simulink library "HEV_Battery_Lib"  (R2024b)
settings: Solver=ode45  StartTime=0.0  StopTime=10.0  RelTol=1e-3  EnableMultiTasking=on
undefined symbols (not defined in the file or in its folder): HEV_Param, Hydride, Kt_Temps, Metal, Nickel
libraries: fl_lib x58, nesl_utility x31, $bdroot x12, Rcecm_lib x6, batteryecm_lib x3, Capacitors_lib x1, spsBatteryLib x1, simulink_extras x1, spsGroundLib x1, spsControlledCurrentSourceLib x1, spsVoltageMeasurementLib x1
(part 1 of 2)
Description:
  | Copyright 2014-2024 The MathWorks, Inc.
settings Model: Creator=smiller  LastModifiedBy=hcseu
settings SolverCC: AlgebraicLoopSolver=TrustRegion
settings DataIOCC: LimitDataPoints=on  SaveFormat=Array  SignalLoggingSaveFormat=ModelDataLogs  ReturnWorkspaceOutputs=off
settings OptimizationCC: ReuseModelBlockBuffer=off  ExpressionDepthLimit=2147483647  LifeSpan=inf
settings DebuggingCC: UnderspecifiedInitializationDetection=Classic  MergeDetectMultiDrivingBlocksExec=none  SolverPrmCheckMsg=warning  FcnCallInpInsideContextMsg=warning  UnconnectedInputMsg=warning  UnconnectedOutputMsg=warning  UnconnectedLineMsg=warning  AllowSymbolicDim=off  StateNameClashWarn=warning  PregeneratedLibrarySubsystemCodeDiagnostic=none  SFUnexpectedBacktrackingDiag=warning  SFNoUnconditionalDefaultTransitionDiag=warning  SFExecutionAtInitializationDiag=none  ArithmeticOperatorsInVariantConditions=warning
settings HardwareCC: ProdBitPerPointer=32  ProdBitPerSizeT=32  ProdBitPerPtrDiffT=32  ProdLargestAtomicFloat=None  ProdIntDivRoundTo=Undefined  ProdEndianess=Unspecified  ProdWordSize=32  ProdHWDeviceType=32-bit Generic
settings ModelReferenceCC: EnableRefExpFcnMdlSchedulingChecks=on  PropagateSignalLabelsOutOfModel=off
settings SFSimCC: SimUseLocalCustomCode=off  CustomCodeUndefinedFunction=UseInterfaceOnly
settings RTWCC: RTWUseLocalCustomCode=off  GPUComputeCapability=3.5  DLArmComputeVersion=19.05
settings CodeAppCC: StateflowObjectComments=on
settings GRTTargetCC: TargetLangStandard=C89/C90 (ANSI)  CombineOutputUpdateFcns=off  GRTInterface=on
settings ConfigComp: CovMetricSettings=dw  CovSaveCumulativeToWorkspaceVar=on  CovSaveSingleToWorkspaceVar=on  CovExternalEMLEnable=off  CovSFcnEnable=off

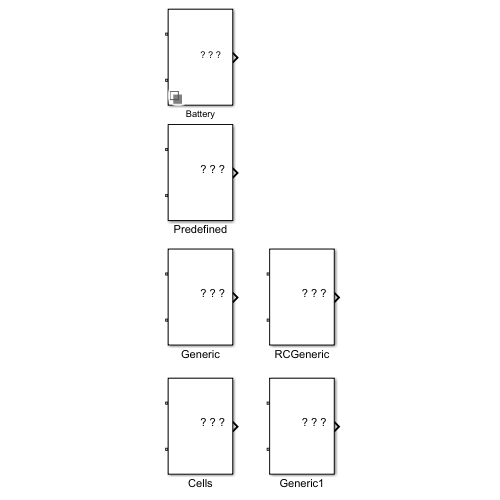
[thumbnail: Simulink's stored preview of the top-level diagram]
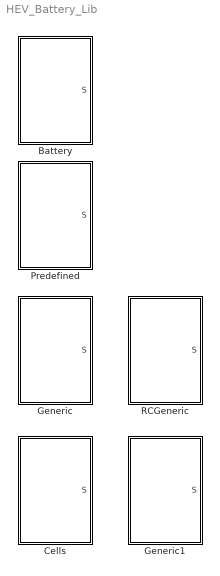
== system HEV_Battery_Lib ==
  Battery : Subsystem  BlockChoice=Predefined  Variant=on  VariantControlMode=label  LabelModeActiveChoice=Predefined
      mask Display:
      | blk = HEVPS_activeVariantBlock(gcb);
      | eval(get_param(blk, 'MaskDisplay'));
  Cells : Subsystem
      mask Display:
      | image(imread('HEV_Battery_Cells_IMAGE.jpg'));
      | port_label('LConn',1,'+');
      | port_label('LConn',2,'-');
      | port_label('output',1,'S');
  Generic : Subsystem
      mask Display:
      | image(imread('HEV_Battery_Custom_IMAGE.jpg'));
      | port_label('LConn',1,'+');
      | port_label('LConn',2,'-');
      | port_label('output',1,'S');
  Generic1 : Subsystem
      mask Display:
      | image(imread('HEV_Battery_Generic_IMAGE.jpg'));
      | port_label('LConn',1,'+');
      | port_label('LConn',2,'-');
      | port_label('output',1,'S');
  Predefined : Subsystem
      mask Display:
      | image(imread('HEV_Battery_Detailed_IMAGE.jpg'));
      | port_label('LConn',1,'+');
      | port_label('LConn',2,'-');
      | port_label('output',1,'S');
  RCGeneric : Subsystem
      mask Display:
      | image(imread('HEV_Battery_GenericRC_IMAGE.jpg'));
      | port_label('LConn',1,'+');
      | port_label('LConn',2,'-');
      | port_label('output',1,'S');

== system HEV_Battery_Lib/Battery ==
  Cells : $bdroot/Cells  SystemSampleTime=-1  VariantControl=Cells  VariantActivationTime=update diagram  AllowFlexibleInterface=on  Latency=0  AutoFrameSizeCalculation=off
  Generic : $bdroot/Generic  SystemSampleTime=-1  VariantControl=Generic  VariantActivationTime=update diagram  AllowFlexibleInterface=on  Latency=0  AutoFrameSizeCalculation=off
  Predefined : $bdroot/Predefined  SystemSampleTime=-1  VariantControl=Predefined  VariantActivationTime=update diagram  AllowFlexibleInterface=on  Latency=0  AutoFrameSizeCalculation=off
  + : PMIOPort  Side=Left
  - : PMIOPort  Port=2  Side=Left
  S : Outport  VectorParamsAs1DForOutWhenUnconnected=off

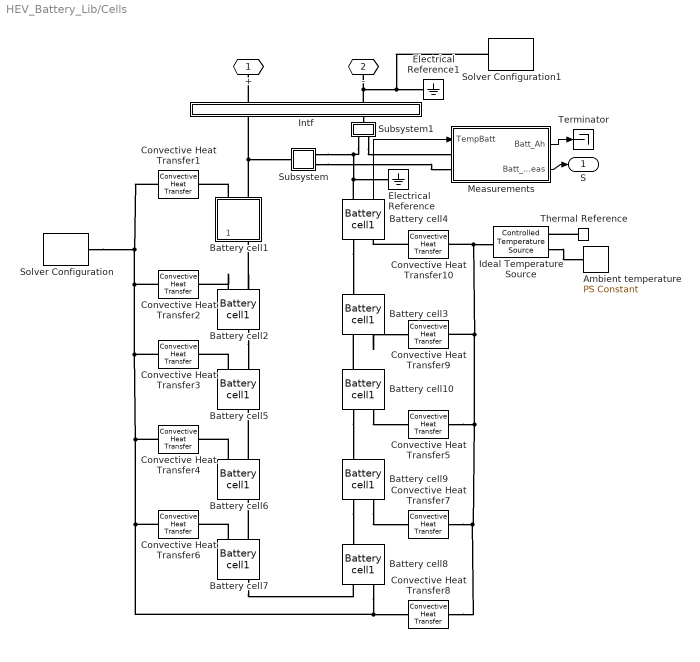
== system HEV_Battery_Lib/Cells ==
  Ambient temperature : fl_lib/Physical Signals/Sources/PS Constant  constant=273+25
  Battery cell1 : Subsystem
      mask Display:
      | % Battery icon
      | plot([1.5 0.4],[0 0])
      | plot(-[0.2 0.9 0.9 1.5],[0 0 -0.8 -0.8])
      | patch(([1 1 -1 -1]*0.15-0.5)*-1,[-1 1 1 -1]*0.4,[0;0;0]);
      | patch(([1 1 -1 -1]*0.15+0.1)*-1,[-1 1 1 -1]*0.9,[0;0;0]);
      | 
      | % Thermal port
      | plot([-0.5,-0.9],[1.2,1.2])
      | plot([-0.5,-0.9],[0.4,0.4])
      | plot([-0.9,-1.5],[0.8,0.8])
      | plot(-0.15*sin(0:2*pi/50:2*pi)-0.85,-0.35*cos(0:2*pi/50:2*pi)+0.8)
      | plot(0.15*sin(0:2*pi/50:pi)-0.55,-0.35*cos(0:2*pi/50:pi)+0.8)
      | 
      | % Plot points to set plot range
      | color('white');plot(1.5,1.5);plot(-1.5,-1.5)
      | 
      | color('red')
      | port_label('LConn',1,'H')
      | port_label('LConn',2,'+')
      | port_label('RConn',1,'-')
  Battery cell{2..10} (9 alike) : $bdroot/Cells/Battery cell1  SystemSampleTime=-1  VariantActivationTime=update diagram  AllowFlexibleInterface=on  Latency=0  AutoFrameSizeCalculation=off
  Convective Heat Transfer{1..10} (10 alike) : fl_lib/Thermal/Thermal Elements/Convective Heat Transfer  thermal_type=foundation.enum.constant_variable.constant  area=HEV_Param.Battery_Cell.Area m^2  heat_tr_coeff=HEV_Param.Battery_Cell.Rtheta W/(m^2 *K)  min_heat_tr_coeff=1e-3 W/(K*m^2)  T_specify=off  T_priority=High  T=0 K  T_nominal_specify=off  T_nominal_value=1  T_nominal_unit=K  Q_specify=off  Q_priority=High  Q=0 J/s  Q_nominal_specify=off  Q_nominal_value=1  Q_nominal_unit=J/s
  Electrical Reference : fl_lib/Electrical/Electrical Elements/Electrical Reference
  Electrical Reference1 : fl_lib/Electrical/Electrical Elements/Electrical Reference
  Ideal Temperature Source : fl_lib/Thermal/Thermal Sources/Controlled Temperature Source
  Intf : Subsystem  mask(Simscape Interface Element){T=100000}
      mask prompts: T "Pole in Transfer Function"
      mask help:
      | Ideal transformer between Simscape circuits.
      |
      | The Voltage across the two terminal pairs are equal and the current flowing through the two branches are equal.
      |
      | The coupling has a transfer function and you need to set the pole in the transfer function.
      mask Display:
      | %color('red');
      | %plot([0.3 0.7],[0.775 0.775]);
      | port_label('LConn', 1,'SPS1')
      | port_label('RConn', 1,'SS1')
      | color('black');
      | %plot([0.3 0.7],[0.225 0.225]);
      | port_label('LConn', 2,'SPS2')
      | port_label('RConn', 2,'SS2')
      | color('green')
      | %text(0.05,0.5,'I Src');
      | color('blue')
      | %text(0.75,0.5,'V Src');
  Measurements : Subsystem
  Solver Configuration : nesl_utility/Solver Configuration  PhysicalDomain=network_engine_domain  SubClassName=solver  LeftPortType=input  RightPortType=generic  Tones=[]  Harmonics=[]  SimulateNoise=off  Profile=off  UseLocalSampling=off  EnableSwitchedLinearOptims=on  FrequencyDomain=off  UseCCode=off  RelTol=0.001  AbsTol=0.001  MinStep=1e-09  ToWorkspace=off  RevertToSquareIcSolve=off  NumHomotopyIterations=100  PhasorMode=off  PhasorModeNumHarmonics=1  ConsistencySolver=NEWTON_XTOL_AFTER_FTOL  IndexReductionMethod=DerivativeReplacement  DoDC=off  ResidualTolerance=1e-09  ConsistencyTolSource=GLOBAL  ConsistencyAbsTol=0.001  ConsistencyRelTol=0.001  ConsistencyTolFactor=0.001  UseLocalSolver=on  LocalSolverChoice=NE_BACKWARD_EULER_ADVANCER  ResolveIndetEquations=on  FunctionEvalNumThread=1  LocalSolverSampleTime=0.001  DoFixedCost=off  MaxNonlinIter=3  MaxModeIter=2  ComputeImpulses=off  ImpulseIterations=2  LinearAlgebra=auto  LinearAlgebraNumThread=0  EquationFormulation=NE_TIME_EF  DelaysMemoryBudget=1024  AutomaticFiltering=on  FilteringTimeConstant=0.001  PartitionStorageMethod=AS_NEEDED  PartitionMemoryBudget=1024  PartitionMethod=ROBUST  MultibodyUseLocalSolver=off  MultibodyLocalSolverChoice=ODE1  MultibodyLocalSolverSampleTime=0.001
  Solver Configuration1 : nesl_utility/Solver Configuration  PhysicalDomain=network_engine_domain  SubClassName=solver  LeftPortType=input  RightPortType=generic  Tones=[]  Harmonics=[]  SimulateNoise=off  Profile=off  UseLocalSampling=off  EnableSwitchedLinearOptims=on  FrequencyDomain=off  UseCCode=off  RelTol=0.001  AbsTol=0.001  MinStep=1e-09  ToWorkspace=off  RevertToSquareIcSolve=off  NumHomotopyIterations=100  PhasorMode=off  PhasorModeNumHarmonics=1  ConsistencySolver=NEWTON_XTOL_AFTER_FTOL  IndexReductionMethod=DerivativeReplacement  DoDC=off  ResidualTolerance=1e-09  ConsistencyTolSource=GLOBAL  ConsistencyAbsTol=0.001  ConsistencyRelTol=0.001  ConsistencyTolFactor=0.001  UseLocalSolver=on  LocalSolverChoice=NE_BACKWARD_EULER_ADVANCER  ResolveIndetEquations=on  FunctionEvalNumThread=1  LocalSolverSampleTime=0.001  DoFixedCost=off  MaxNonlinIter=3  MaxModeIter=2  ComputeImpulses=off  ImpulseIterations=2  LinearAlgebra=auto  LinearAlgebraNumThread=0  EquationFormulation=NE_TIME_EF  DelaysMemoryBudget=1024  AutomaticFiltering=on  FilteringTimeConstant=0.001  PartitionStorageMethod=AS_NEEDED  PartitionMemoryBudget=1024  PartitionMethod=ROBUST  MultibodyUseLocalSolver=off  MultibodyLocalSolverChoice=ODE1  MultibodyLocalSolverSampleTime=0.001
  Subsystem : Subsystem
      mask Display: disp('S')
  Subsystem1 : Subsystem
      mask Display: disp('S');
  Terminator : Terminator
  Thermal Reference : fl_lib/Thermal/Thermal Elements/Thermal Reference
  + : PMIOPort  Side=Left
  - : PMIOPort  Port=2  Side=Left
  S : Outport  VectorParamsAs1DForOutWhenUnconnected=off
  wires:
  Measurements/2(Batt_Meas) -> S/1
  Measurements/1(Batt_Ah) -> Terminator/1
  Battery cell4/1 -> Measurements/1(TempBatt)
  connections:
  -/RConn1 -- Solver Configuration1/RConn1 -- Electrical Reference1/LConn1 -- Intf/RConn2
  Intf/RConn1 -- +/RConn1
  Intf/LConn2 -- Subsystem1/LConn1
  Subsystem1/RConn2 -- Measurements/LConn1
  Subsystem1/RConn1 -- Subsystem/RConn2 -- Battery cell4/RConn1 -- Electrical Reference/LConn1
  Subsystem/RConn1 -- Measurements/LConn2
  Battery cell1/LConn2 -- Subsystem/LConn1 -- Intf/LConn1
  Battery cell3/LConn1 -- Convective Heat Transfer9/RConn1
  Battery cell4/LConn2 -- Battery cell3/RConn1
  Battery cell2/LConn1 -- Convective Heat Transfer2/RConn1
  Battery cell1/LConn1 -- Convective Heat Transfer1/RConn1
  Ideal Temperature Source/RConn1 -- Ambient temperature/RConn1
  Thermal Reference/LConn1 -- Ideal Temperature Source/RConn2
  Battery cell10/LConn1 -- Convective Heat Transfer5/RConn1
  Battery cell10/RConn1 -- Battery cell3/LConn2
  Battery cell2/LConn2 -- Battery cell1/RConn1
  Convective Heat Transfer10/RConn1 -- Battery cell4/LConn1
  Convective Heat Transfer5/LConn1 -- Convective Heat Transfer7/LConn1 -- Convective Heat Transfer8/LConn1 -- Convective Heat Transfer9/LConn1 -- Convective Heat Transfer10/LConn1 -- Ideal Temperature Source/LConn1
  Battery cell6/LConn2 -- Battery cell5/RConn1
  Battery cell7/LConn2 -- Battery cell6/RConn1
  Battery cell9/LConn2 -- Battery cell8/RConn1
  Battery cell10/LConn2 -- Battery cell9/RConn1
  Battery cell7/RConn1 -- Battery cell8/LConn2
  Battery cell2/RConn1 -- Battery cell5/LConn2
  Battery cell5/LConn1 -- Convective Heat Transfer3/RConn1
  Battery cell6/LConn1 -- Convective Heat Transfer4/RConn1
  Battery cell7/LConn1 -- Convective Heat Transfer6/RConn1
  Battery cell9/LConn1 -- Convective Heat Transfer7/RConn1
  Convective Heat Transfer3/LConn1 -- Convective Heat Transfer4/LConn1 -- Convective Heat Transfer8/RConn1 -- Battery cell8/LConn1 -- Convective Heat Transfer6/LConn1 -- Convective Heat Transfer2/LConn1 -- Solver Configuration/RConn1 -- Convective Heat Transfer1/LConn1

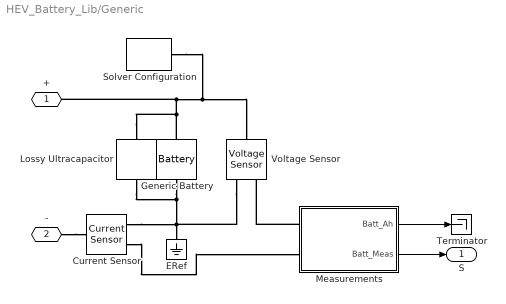
== system HEV_Battery_Lib/Generic ==
  Current Sensor : fl_lib/Electrical/Electrical Sensors/Current Sensor
  ERef : fl_lib/Electrical/Electrical Elements/Electrical Reference
  Generic Battery : batteryecm_lib/Battery  Vnom=HEV_Param.Battery_Sys.Nominal_Voltage V  prm_dir=1  R1_dis=2 Ohm  R1_ch=2 Ohm  R1=HEV_Param.Battery_Sys.Internal_Resistance Ohm  prm_AH=2  AH=HEV_Param.Battery_Sys.Rated_Capacity hr*A  V1=HEV_Param.Battery_Sys.Expn_Voltage V  AH1=HEV_Param.Battery_Sys.Expn_Charge hr*A  prm_R2=1  R2=2e+3 Ohm  Tmeas=298.15 K  charge_measurement_port=simscape.enum.battery.enable.no  prm_dyn=1  Rp1=0.005 Ohm  tau1=30 s  Rp2=0.005 Ohm  tau2=30 s  Rp3=0.005 Ohm  tau3=30 s  Rp4=0.005 Ohm  tau4=30 s  Rp5=0.005 Ohm  tau5=30 s  prm_fade=1  N_fade=100  AH_fade=45 hr*A  R1_fade=2.02 Ohm  R1_ch_fade=2.02 Ohm  V1_fade=10.35 V  prm_age=1  prm_age_OCV=1  OCV_age=0.9  SOC_age=60  Tmeas_age=298.15 K  delta_time_age_vec=[0] d  temperature_age_vec=[273] K  OCV_scaling_age=2.2134e6  OCV_offset_age=1.632e6  temp_exp_age=0.515833569 V  t_exp_age=0.75  Vnom_T2=12 V  R1_T2=2.2 Ohm  R1_T2_dis=2.2 Ohm  R1_T2_ch=2.2 Ohm  V1_T2=11.4 V  R2_T2=2200 Ohm  Rp1_T2=0.005 Ohm  tau1_T2=30 s  Rp2_T2=0.005 Ohm  tau2_T2=30 s  Rp3_T2=0.005 Ohm  tau3_T2=30 s  Rp4_T2=0.005 Ohm  tau4_T2=30 s  Rp5_T2=0.005 Ohm  tau5_T2=30 s  Tmeas2=273.15 K  thermal_port=simscape.enum.thermaleffects.omit  thermal_mass=30000 J/K  i_specify=off  i_priority=None  i=0 A  i_nominal_specify=off  i_nominal_value=1  i_nominal_unit=A  v_specify=off  v_priority=None  v=0 V  v_nominal_specify=off  v_nominal_value=1  v_nominal_unit=V  charge_specify=on  charge_priority=High  charge=HEV_Param.Battery_Sys.Initial_Charge hr*A  charge_nominal_specify=off  charge_nominal_value=1  charge_nominal_unit=A*hr  num_cycles_specify=off  num_cycles_priority=High  num_cycles=0  num_cycles_nominal_specify=off  num_cycles_nominal_value=1  num_cycles_nominal_unit=1  temperature_specify=off  temperature_priority=High  temperature=298.15 K  temperature_nominal_specify=off  temperature_nominal_value=1  temperature_nominal_unit=K
  Lossy Ultracapacitor : Capacitors_lib/Lossy Ultracapacitor  C0=HEV_Param.UltraCapacitor.Nominal_Capacitance F  Cv=HEV_Param.UltraCapacitor.Rate_C_V F/V  R=HEV_Param.UltraCapacitor.Series_R Ohm  Rd=HEV_Param.UltraCapacitor.Self_Discharge_R Ohm  i_specify=off  i_priority=High  i=0 A  i_nominal_specify=off  i_nominal_value=1  i_nominal_unit=A  vc_specify=off  vc_priority=High  vc=0 V  vc_nominal_specify=off  vc_nominal_value=1  vc_nominal_unit=V
      settings: InternalSimscapePortConfiguration="{\"Bottom\":[],\"Left\":[{\"id\":\"p\",\"label\":\"+\",\"type\":\"foundation.electrical.electrical\"}],\"Right\":[{\"id\":\"n\",\"label\":\"-\",\"type\":\"foundation.electrical.electrical\"}],\"Top\":[]}"
  Measurements : Subsystem
  Solver Configuration : nesl_utility/Solver Configuration  PhysicalDomain=network_engine_domain  SubClassName=solver  LeftPortType=input  RightPortType=generic  Tones=[]  Harmonics=[]  SimulateNoise=off  Profile=off  UseLocalSampling=off  EnableSwitchedLinearOptims=on  FrequencyDomain=off  UseCCode=off  RelTol=0.001  AbsTol=0.001  MinStep=1e-09  ToWorkspace=off  RevertToSquareIcSolve=off  NumHomotopyIterations=100  PhasorMode=off  PhasorModeNumHarmonics=1  ConsistencySolver=NEWTON_XTOL_AFTER_FTOL  IndexReductionMethod=DerivativeReplacement  DoDC=off  ResidualTolerance=1e-09  ConsistencyTolSource=GLOBAL  ConsistencyAbsTol=0.001  ConsistencyRelTol=0.001  ConsistencyTolFactor=0.001  UseLocalSolver=off  LocalSolverChoice=NE_BACKWARD_EULER_ADVANCER  ResolveIndetEquations=on  FunctionEvalNumThread=1  LocalSolverSampleTime=0.001  DoFixedCost=off  MaxNonlinIter=3  MaxModeIter=2  ComputeImpulses=off  ImpulseIterations=2  LinearAlgebra=auto  LinearAlgebraNumThread=0  EquationFormulation=NE_TIME_EF  DelaysMemoryBudget=1024  AutomaticFiltering=on  FilteringTimeConstant=0.001  PartitionStorageMethod=AS_NEEDED  PartitionMemoryBudget=1024  PartitionMethod=ROBUST  MultibodyUseLocalSolver=off  MultibodyLocalSolverChoice=ODE1  MultibodyLocalSolverSampleTime=0.001
  Terminator : Terminator
  Voltage Sensor : fl_lib/Electrical/Electrical Sensors/Voltage Sensor
  + : PMIOPort  Side=Left
  - : PMIOPort  Port=2  Side=Left
  S : Outport  VectorParamsAs1DForOutWhenUnconnected=off
  wires:
  Measurements/2(Batt_Meas) -> S/1
  Measurements/1(Batt_Ah) -> Terminator/1
  connections:
  -/RConn1 -- Current Sensor/LConn1
  Current Sensor/RConn1 -- Measurements/LConn2
  Lossy Ultracapacitor/RConn1 -- Current Sensor/RConn2 -- ERef/LConn1 -- Voltage Sensor/RConn2 -- Generic Battery/RConn1
  Lossy Ultracapacitor/LConn1 -- +/RConn1 -- Solver Configuration/RConn1 -- Voltage Sensor/LConn1 -- Generic Battery/LConn1
  Measurements/LConn1 -- Voltage Sensor/RConn1

== system HEV_Battery_Lib/Generic1 ==
  Current Sensor : fl_lib/Electrical/Electrical Sensors/Current Sensor
  Electrical Reference : fl_lib/Electrical/Electrical Elements/Electrical Reference
  Generic Battery : batteryecm_lib/Battery  Vnom=HEV_Param.Battery_Sys.Nominal_Voltage V  prm_dir=1  R1_dis=2 Ohm  R1_ch=2 Ohm  R1=HEV_Param.Battery_Sys.Internal_Resistance Ohm  prm_AH=2  AH=HEV_Param.Battery_Sys.Rated_Capacity hr*A  V1=HEV_Param.Battery_Sys.Expn_Voltage V  AH1=HEV_Param.Battery_Sys.Expn_Charge hr*A  prm_R2=1  R2=2e+3 Ohm  Tmeas=298.15 K  charge_measurement_port=simscape.enum.battery.enable.no  prm_dyn=1  Rp1=0.005 Ohm  tau1=30 s  Rp2=0.005 Ohm  tau2=30 s  Rp3=0.005 Ohm  tau3=30 s  Rp4=0.005 Ohm  tau4=30 s  Rp5=0.005 Ohm  tau5=30 s  prm_fade=1  N_fade=100  AH_fade=45 hr*A  R1_fade=2.02 Ohm  R1_ch_fade=2.02 Ohm  V1_fade=10.35 V  prm_age=1  prm_age_OCV=1  OCV_age=0.9  SOC_age=60  Tmeas_age=298.15 K  delta_time_age_vec=[0] d  temperature_age_vec=[273] K  OCV_scaling_age=2.2134e6  OCV_offset_age=1.632e6  temp_exp_age=0.515833569 V  t_exp_age=0.75  Vnom_T2=12 V  R1_T2=2.2 Ohm  R1_T2_dis=2.2 Ohm  R1_T2_ch=2.2 Ohm  V1_T2=11.4 V  R2_T2=2200 Ohm  Rp1_T2=0.005 Ohm  tau1_T2=30 s  Rp2_T2=0.005 Ohm  tau2_T2=30 s  Rp3_T2=0.005 Ohm  tau3_T2=30 s  Rp4_T2=0.005 Ohm  tau4_T2=30 s  Rp5_T2=0.005 Ohm  tau5_T2=30 s  Tmeas2=273.15 K  thermal_port=simscape.enum.thermaleffects.omit  thermal_mass=30000 J/K  i_specify=off  i_priority=None  i=0 A  i_nominal_specify=off  i_nominal_value=1  i_nominal_unit=A  v_specify=off  v_priority=None  v=0 V  v_nominal_specify=off  v_nominal_value=1  v_nominal_unit=V  charge_specify=on  charge_priority=High  charge=HEV_Param.Battery_Sys.Initial_Charge hr*A  charge_nominal_specify=off  charge_nominal_value=1  charge_nominal_unit=A*hr  num_cycles_specify=off  num_cycles_priority=High  num_cycles=0  num_cycles_nominal_specify=off  num_cycles_nominal_value=1  num_cycles_nominal_unit=1  temperature_specify=off  temperature_priority=High  temperature=298.15 K  temperature_nominal_specify=off  temperature_nominal_value=1  temperature_nominal_unit=K
  Measurements : Subsystem
  Terminator : Terminator
  Voltage Sensor1 : fl_lib/Electrical/Electrical Sensors/Voltage Sensor
  + : PMIOPort  Side=Left
  - : PMIOPort  Port=2  Side=Left
  S : Outport  VectorParamsAs1DForOutWhenUnconnected=off
  wires:
  Measurements/2(Batt_Meas) -> S/1
  Measurements/1(Batt_Ah) -> Terminator/1
  connections:
  -/RConn1 -- Current Sensor/LConn1
  Measurements/LConn2 -- Current Sensor/RConn1
  Current Sensor/RConn2 -- Electrical Reference/LConn1 -- Generic Battery/RConn1 -- Voltage Sensor1/RConn2
  +/RConn1 -- Generic Battery/LConn1 -- Voltage Sensor1/LConn1
  Measurements/LConn1 -- Voltage Sensor1/RConn1

== system HEV_Battery_Lib/Predefined ==
  Battery : spsBatteryLib/Battery  BatType=Nickel-Metal-Hydride  NomV=HEV_Param.Battery_Det.Nominal_Voltage  NomQ=HEV_Param.Battery_Det.Rated_Capacity  SOC=HEV_Param.Battery_Det.Initial_SOC  Batt_Tr=30  PresetModel=on  MaxQ=8.7231  MinV=150  FullV=235.5932  Dis_rate=1.62  R=0.24691  Normal_OP=7.7885  expZone="[216.9492          1.62]"
  Electrical Reference : fl_lib/Electrical/Electrical Elements/Electrical Reference
  GF1 : Subsystem
      mask Display: disp('GF')
  Ground : spsGroundLib/Ground  LConnTagsString=a
  Intf : Subsystem  mask(Power Systems ST - Simscape Interface Element){T=100000}
      mask prompts: T "Pole in Transfer Function"
      mask help:
      | Ideal transformer between a Simscape Power Systems ST circuit and a Simscape circuit.
      |
      | The Voltage across the two terminal pairs are equal and the current flowing through the two branches are equal.
      |
      | The coupling has a transfer function and you need to set the pole in the transfer function.
      mask Display:
      | %color('red');
      | %plot([0.3 0.7],[0.775 0.775]);
      | port_label('LConn', 1,'SPS1')
      | port_label('RConn', 1,'SS1')
      | color('black');
      | %plot([0.3 0.7],[0.225 0.225]);
      | port_label('LConn', 2,'SPS2')
      | port_label('RConn', 2,'SS2')
      | color('green')
      | %text(0.05,0.5,'I Src');
      | color('blue')
      | %text(0.75,0.5,'V Src');
  Solver Configuration : nesl_utility/Solver Configuration  PhysicalDomain=network_engine_domain  SubClassName=solver  LeftPortType=input  RightPortType=generic  Tones=[]  Harmonics=[]  SimulateNoise=off  Profile=off  UseLocalSampling=off  EnableSwitchedLinearOptims=on  FrequencyDomain=off  UseCCode=off  RelTol=0.001  AbsTol=0.001  MinStep=1e-09  ToWorkspace=off  RevertToSquareIcSolve=off  NumHomotopyIterations=100  PhasorMode=off  PhasorModeNumHarmonics=1  ConsistencySolver=NEWTON_XTOL_AFTER_FTOL  IndexReductionMethod=DerivativeReplacement  DoDC=off  ResidualTolerance=1e-09  ConsistencyTolSource=GLOBAL  ConsistencyAbsTol=0.001  ConsistencyRelTol=0.001  ConsistencyTolFactor=0.001  UseLocalSolver=off  LocalSolverChoice=NE_BACKWARD_EULER_ADVANCER  ResolveIndetEquations=on  FunctionEvalNumThread=1  LocalSolverSampleTime=0.001  DoFixedCost=off  MaxNonlinIter=3  MaxModeIter=2  ComputeImpulses=off  ImpulseIterations=2  LinearAlgebra=auto  LinearAlgebraNumThread=0  EquationFormulation=NE_TIME_EF  DelaysMemoryBudget=1024  AutomaticFiltering=on  FilteringTimeConstant=0.001  PartitionStorageMethod=AS_NEEDED  PartitionMemoryBudget=1024  PartitionMethod=ROBUST  MultibodyUseLocalSolver=off  MultibodyLocalSolverChoice=ODE1  MultibodyLocalSolverSampleTime=0.001
  + : PMIOPort  Side=Left
  - : PMIOPort  Port=2  Side=Left
  S : Outport  VectorParamsAs1DForOutWhenUnconnected=off
  wires:
  Battery/1 -> GF1/1(In1)
  GF1/1(Out1) -> S/1
  connections:
  Intf/RConn2 -- Solver Configuration/RConn1 -- Electrical Reference/LConn1 -- -/RConn1
  Intf/LConn2 -- Battery/LConn2 -- Ground/LConn1
  Battery/LConn1 -- Intf/LConn1
  +/RConn1 -- Intf/RConn1

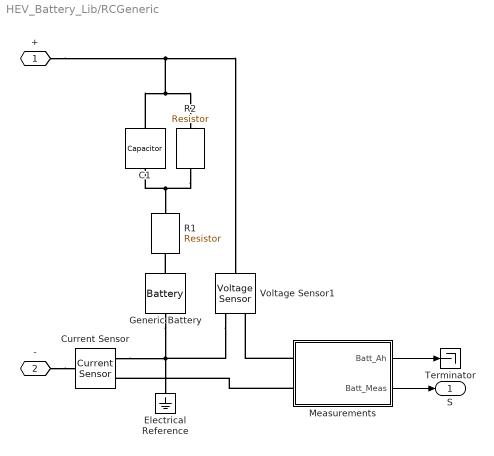
== system HEV_Battery_Lib/RCGeneric ==
  C1 : fl_lib/Electrical/Electrical Elements/Capacitor  c=HEV_Param.Battery_Sys.C1.Capacitance F  r=HEV_Param.Battery_Sys.C1.Series_Resistance Ohm  g=0 1/Ohm  i_specify=off  i_priority=High  i=0 A  i_nominal_specify=off  i_nominal_value=1  i_nominal_unit=A  v_specify=off  v_priority=High  v=0 V  v_nominal_specify=off  v_nominal_value=1  v_nominal_unit=V  vc_specify=on  vc_priority=High  vc=HEV_Param.Battery_Sys.C1.Initial_Voltage V  vc_nominal_specify=off  vc_nominal_value=1  vc_nominal_unit=V
  Current Sensor : fl_lib/Electrical/Electrical Sensors/Current Sensor
  Electrical Reference : fl_lib/Electrical/Electrical Elements/Electrical Reference
  Generic Battery : batteryecm_lib/Battery  Vnom=HEV_Param.Battery_Sys.Nominal_Voltage V  prm_dir=1  R1_dis=2 Ohm  R1_ch=2 Ohm  R1=HEV_Param.Battery_Sys.Internal_Resistance Ohm  prm_AH=2  AH=HEV_Param.Battery_Sys.Rated_Capacity hr*A  V1=HEV_Param.Battery_Sys.Expn_Voltage V  AH1=HEV_Param.Battery_Sys.Expn_Charge hr*A  prm_R2=1  R2=2e+3 Ohm  Tmeas=298.15 K  charge_measurement_port=simscape.enum.battery.enable.no  prm_dyn=1  Rp1=0.005 Ohm  tau1=30 s  Rp2=0.005 Ohm  tau2=30 s  Rp3=0.005 Ohm  tau3=30 s  Rp4=0.005 Ohm  tau4=30 s  Rp5=0.005 Ohm  tau5=30 s  prm_fade=1  N_fade=100  AH_fade=45 hr*A  R1_fade=2.02 Ohm  R1_ch_fade=2.02 Ohm  V1_fade=10.35 V  prm_age=1  prm_age_OCV=1  OCV_age=0.9  SOC_age=60  Tmeas_age=298.15 K  delta_time_age_vec=[0] d  temperature_age_vec=[273] K  OCV_scaling_age=2.2134e6  OCV_offset_age=1.632e6  temp_exp_age=0.515833569 V  t_exp_age=0.75  Vnom_T2=12 V  R1_T2=2.2 Ohm  R1_T2_dis=2.2 Ohm  R1_T2_ch=2.2 Ohm  V1_T2=11.4 V  R2_T2=2200 Ohm  Rp1_T2=0.005 Ohm  tau1_T2=30 s  Rp2_T2=0.005 Ohm  tau2_T2=30 s  Rp3_T2=0.005 Ohm  tau3_T2=30 s  Rp4_T2=0.005 Ohm  tau4_T2=30 s  Rp5_T2=0.005 Ohm  tau5_T2=30 s  Tmeas2=273.15 K  thermal_port=simscape.enum.thermaleffects.omit  thermal_mass=30000 J/K  i_specify=off  i_priority=None  i=0 A  i_nominal_specify=off  i_nominal_value=1  i_nominal_unit=A  v_specify=off  v_priority=None  v=0 V  v_nominal_specify=off  v_nominal_value=1  v_nominal_unit=V  charge_specify=on  charge_priority=High  charge=HEV_Param.Battery_Sys.Initial_Charge hr*A  charge_nominal_specify=off  charge_nominal_value=1  charge_nominal_unit=A*hr  num_cycles_specify=off  num_cycles_priority=High  num_cycles=0  num_cycles_nominal_specify=off  num_cycles_nominal_value=1  num_cycles_nominal_unit=1  temperature_specify=off  temperature_priority=High  temperature=298.15 K  temperature_nominal_specify=off  temperature_nominal_value=1  temperature_nominal_unit=K
  Measurements : Subsystem
  R1 : fl_lib/Electrical/Electrical Elements/Resistor  R=HEV_Param.Battery_Sys.R1 Ohm  i_specify=off  i_priority=High  i=0 A  i_nominal_specify=off  i_nominal_value=1  i_nominal_unit=A  v_specify=off  v_priority=High  v=0 V  v_nominal_specify=off  v_nominal_value=1  v_nominal_unit=V
  R2 : fl_lib/Electrical/Electrical Elements/Resistor  R=HEV_Param.Battery_Sys.R2 Ohm  i_specify=off  i_priority=High  i=0 A  i_nominal_specify=off  i_nominal_value=1  i_nominal_unit=A  v_specify=off  v_priority=High  v=0 V  v_nominal_specify=off  v_nominal_value=1  v_nominal_unit=V
  Terminator : Terminator
  Voltage Sensor1 : fl_lib/Electrical/Electrical Sensors/Voltage Sensor
  + : PMIOPort  Side=Left
  - : PMIOPort  Port=2  Side=Left
  S : Outport  VectorParamsAs1DForOutWhenUnconnected=off
  wires:
  Measurements/1(Batt_Ah) -> Terminator/1
  Measurements/2(Batt_Meas) -> S/1
  connections:
  Measurements/LConn1 -- Voltage Sensor1/RConn1
  +/RConn1 -- Voltage Sensor1/LConn1 -- R2/LConn1 -- C1/LConn1
  Voltage Sensor1/RConn2 -- Generic Battery/RConn1 -- Electrical Reference/LConn1 -- Current Sensor/RConn2
  Measurements/LConn2 -- Current Sensor/RConn1
  -/RConn1 -- Current Sensor/LConn1
  R2/RConn1 -- R1/LConn1 -- C1/RConn1
  Generic Battery/LConn1 -- R1/RConn1

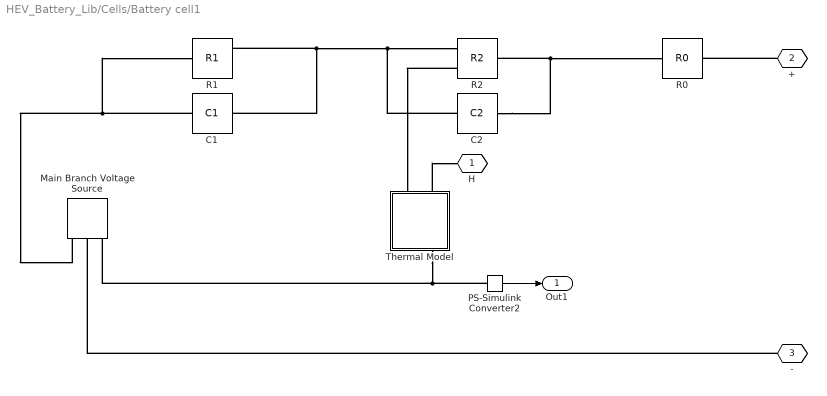
== system HEV_Battery_Lib/Cells/Battery cell1 ==
  C1 : Rcecm_lib/C1  Tau1=HEV_Param.Battery_Cell.Tau1 s  Cmin=1e-6 F  R1=HEV_Param.Battery_Cell.R1 Ohm
      settings: InternalSimscapePortConfiguration="{\"Bottom\":[],\"Left\":[{\"id\":\"p\",\"label\":\"+\",\"type\":\"foundation.electrical.electrical\"}],\"Right\":[{\"id\":\"n\",\"label\":\"-\",\"type\":\"foundation.electrical.electrical\"}],\"Top\":[]}"
  C2 : Rcecm_lib/C2  C2=HEV_Param.Battery_Cell.C2 F  i_specify=off  i_priority=None  i=0 A  i_nominal_specify=off  i_nominal_value=1  i_nominal_unit=A  q_specify=off  q_priority=None  q=0 C  q_nominal_specify=off  q_nominal_value=1  q_nominal_unit=C
      settings: InternalSimscapePortConfiguration="{\"Bottom\":[],\"Left\":[{\"id\":\"p\",\"label\":\"+\",\"type\":\"foundation.electrical.electrical\"}],\"Right\":[{\"id\":\"n\",\"label\":\"-\",\"type\":\"foundation.electrical.electrical\"}],\"Top\":[]}"
  Main Branch Voltage Source : Rcecm_lib/Main Branch Voltage Source  Em0=HEV_Param.Battery_Cell.Emo V  Ke=0.0006 V/K  Cbat=HEV_Param.Battery_Cell.Rated_Capacity Ah  Qinit=0 A*s  Rint=1e-3 Ohm
      settings: InternalSimscapePortConfiguration="{\"Bottom\":[],\"Left\":[{\"id\":\"p\",\"label\":\"+\",\"type\":\"foundation.electrical.electrical\"},{\"id\":\"n\",\"label\":\"-\",\"type\":\"foundation.electrical.electrical\"},{\"id\":\"T\",\"label\":\"Temperature input\",\"type\":\"input\"}],\"Right\":[{\"id\":\"SOC\",\"label\":\"State of charge\",\"type\":\"output\"}],\"Top\":[]}"
  PS-Simulink Converter2 : nesl_utility/PS-Simulink Converter  PhysicalDomain=network_engine_domain  SubClassName=ps_output  LeftPortType=input  RightPortType=output  PseudoPeriodic=off  Frequencies=[]  VectorFormat=inherit  Unit=inherit  AffineConversion=off
  R0 : Rcecm_lib/R0  R00=HEV_Param.Battery_Cell.R0 Ohm
      settings: InternalSimscapePortConfiguration="{\"Bottom\":[],\"Left\":[{\"id\":\"p\",\"label\":\"+\",\"type\":\"foundation.electrical.electrical\"}],\"Right\":[{\"id\":\"n\",\"label\":\"-\",\"type\":\"foundation.electrical.electrical\"}],\"Top\":[]}"
  R1 : Rcecm_lib/R1  R10=HEV_Param.Battery_Cell.R1 Ohm
      settings: InternalSimscapePortConfiguration="{\"Bottom\":[],\"Left\":[{\"id\":\"p\",\"label\":\"+\",\"type\":\"foundation.electrical.electrical\"},{\"id\":\"R1\",\"label\":\"R1\",\"type\":\"output\"}],\"Right\":[{\"id\":\"n\",\"label\":\"-\",\"type\":\"foundation.electrical.electrical\"}],\"Top\":[]}"
  R2 : Rcecm_lib/R2  R2=HEV_Param.Battery_Cell.R2 Ohm
      settings: InternalSimscapePortConfiguration="{\"Bottom\":[],\"Left\":[{\"id\":\"p\",\"label\":\"+\",\"type\":\"foundation.electrical.electrical\"}],\"Right\":[{\"id\":\"n\",\"label\":\"-\",\"type\":\"foundation.electrical.electrical\"},{\"id\":\"pow\",\"label\":\"POW\",\"type\":\"output\"}],\"Top\":[]}"
  Thermal Model : Subsystem
  H : PMIOPort  Tag=PMCPort  Side=Left
  + : PMIOPort  Tag=PMCPort  Port=2  Side=Left
  - : PMIOPort  Tag=PMCPort  Port=3  Side=Right
  Out1 : Outport
  wires:
  PS-Simulink Converter2/1 -> Out1/1
  connections:
  +/RConn1 -- R0/LConn1
  C1/RConn1 -- Main Branch Voltage Source/LConn1 -- R1/RConn1
  C2/LConn1 -- R0/RConn1 -- R2/LConn1
  Thermal Model/LConn2 -- H/RConn1
  C1/LConn1 -- R1/LConn1 -- C2/RConn1 -- R2/RConn1
  R2/RConn2 -- Thermal Model/LConn1
  -/RConn1 -- Main Branch Voltage Source/LConn2
  Thermal Model/RConn2 -- Main Branch Voltage Source/LConn3 -- PS-Simulink Converter2/LConn1

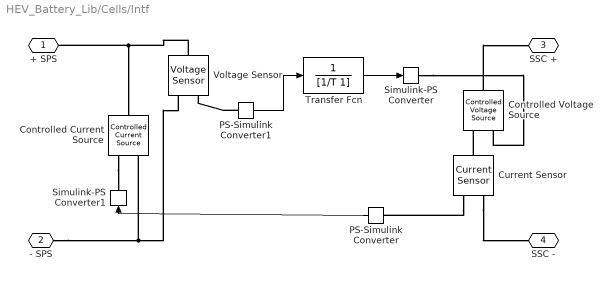
== system HEV_Battery_Lib/Cells/Intf ==
  Controlled Voltage Source : fl_lib/Electrical/Electrical Sources/Controlled Voltage Source
  Controlled Current Source : fl_lib/Electrical/Electrical Sources/Controlled Current Source
  Current Sensor : fl_lib/Electrical/Electrical Sensors/Current Sensor
  PS-Simulink Converter : nesl_utility/PS-Simulink Converter  PhysicalDomain=network_engine_domain  SubClassName=ps_output  LeftPortType=input  RightPortType=output  PseudoPeriodic=off  Frequencies=[]  VectorFormat=1-D array  Unit=A  AffineConversion=off
  PS-Simulink Converter1 : nesl_utility/PS-Simulink Converter  PhysicalDomain=network_engine_domain  SubClassName=ps_output  LeftPortType=input  RightPortType=output  PseudoPeriodic=off  Frequencies=[]  VectorFormat=1-D array  Unit=V  AffineConversion=off
  Simulink-PS Converter : nesl_utility/Simulink-PS Converter  PhysicalDomain=network_engine_domain  SubClassName=ps_input  LeftPortType=input  RightPortType=output  PseudoPeriodic=off  Frequencies=[]  NoiseDistribution=none  NoiseParameters=[]  Unit=V  AffineConversion=off  FilteringAndDerivatives=zero  SimscapeFilterOrder=1  InputFilterTimeConstant=0.005  UdotUserProvided=0
  Simulink-PS Converter1 : nesl_utility/Simulink-PS Converter  PhysicalDomain=network_engine_domain  SubClassName=ps_input  LeftPortType=input  RightPortType=output  PseudoPeriodic=off  Frequencies=[]  NoiseDistribution=none  NoiseParameters=[]  Unit=A  AffineConversion=off  FilteringAndDerivatives=zero  SimscapeFilterOrder=1  InputFilterTimeConstant=0.005  UdotUserProvided=0
  Transfer Fcn : TransferFcn  Denominator=[1/T 1]
  Voltage Sensor : fl_lib/Electrical/Electrical Sensors/Voltage Sensor
  + SPS : PMIOPort  Side=Left
  - SPS : PMIOPort  Port=2  Side=Left
  SSC + : PMIOPort  Port=3  Side=Right
  SSC - : PMIOPort  Port=4  Side=Right
  wires:
  PS-Simulink Converter1/1 -> Transfer Fcn/1
  Transfer Fcn/1 -> Simulink-PS Converter/1
  PS-Simulink Converter/1 -> Simulink-PS Converter1/1
  connections:
  Controlled Current Source/RConn1 -- Simulink-PS Converter1/RConn1
  PS-Simulink Converter1/LConn1 -- Voltage Sensor/RConn1
  Voltage Sensor/LConn1 -- + SPS/RConn1 -- Controlled Current Source/LConn1
  Current Sensor/RConn2 -- SSC -/RConn1
  Voltage Sensor/RConn2 -- - SPS/RConn1 -- Controlled Current Source/RConn2
  Current Sensor/RConn1 -- PS-Simulink Converter/LConn1
  Simulink-PS Converter/RConn1 -- Controlled Voltage Source/RConn1
  Current Sensor/LConn1 -- Controlled Voltage Source/RConn2
  Controlled Voltage Source/LConn1 -- SSC +/RConn1

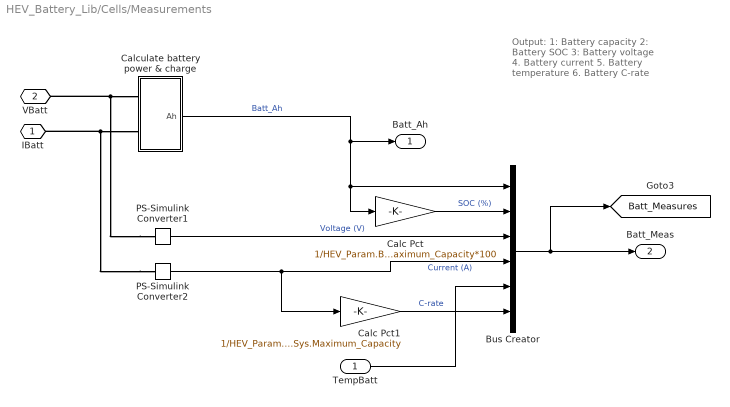
== system HEV_Battery_Lib/Cells/Measurements ==
  note: Output:
      | 1: Battery capacity
      | 2: Battery SOC
      | 3: Battery voltage
      | 4. Battery current
      | 5. Battery temperature
      | 6. Battery C-rate
  TempBatt : Inport
  Bus Creator : BusCreator  Inputs=6
  Calc Pct : Gain  Gain=1/HEV_Param.Battery_Sys.Maximum_Capacity*100
  Calc Pct1 : Gain  Gain=1/HEV_Param.Battery_Sys.Maximum_Capacity
  Calculate battery power & charge : Subsystem
  PS-Simulink Converter1 : nesl_utility/PS-Simulink Converter  PhysicalDomain=network_engine_domain  SubClassName=ps_output  LeftPortType=input  RightPortType=output  PseudoPeriodic=off  Frequencies=[]  VectorFormat=1-D array  Unit=V  AffineConversion=off
  PS-Simulink Converter2 : nesl_utility/PS-Simulink Converter  PhysicalDomain=network_engine_domain  SubClassName=ps_output  LeftPortType=input  RightPortType=output  PseudoPeriodic=off  Frequencies=[]  VectorFormat=1-D array  Unit=A  AffineConversion=off
  IBatt : PMIOPort  Side=Left
  VBatt : PMIOPort  Port=2  Side=Left
  Batt_Ah : Outport  VectorParamsAs1DForOutWhenUnconnected=off
  Batt_Meas : Outport  Port=2  VectorParamsAs1DForOutWhenUnconnected=off
  tag scope: Batt_Measures=global
  wires:
  Bus Creator/1 -> [Batt_Measures], Batt_Meas/1
  PS-Simulink Converter1/1 -> Bus Creator/3  "Voltage (V)"
  Calc Pct/1 -> Bus Creator/2  "SOC (%)"
  Calculate battery power & charge/1(Ah) -> Batt_Ah/1, Calc Pct/1, Bus Creator/1  "Batt_Ah"
  TempBatt/1 -> Bus Creator/5
  PS-Simulink Converter2/1 -> Calc Pct1/1, Bus Creator/4  "Current (A)"
  Calc Pct1/1 -> Bus Creator/6  "C-rate"
  connections:
  PS-Simulink Converter2/LConn1 -- IBatt/RConn1 -- Calculate battery power & charge/LConn2
  PS-Simulink Converter1/LConn1 -- VBatt/RConn1 -- Calculate battery power & charge/LConn1

== system HEV_Battery_Lib/Cells/Subsystem ==
  Voltage Sensor1 : fl_lib/Electrical/Electrical Sensors/Voltage Sensor
  Conn1 : PMIOPort  Side=Right
  Conn2 : PMIOPort  Port=2  Side=Left
  Conn3 : PMIOPort  Port=3  Side=Right
  connections:
  Conn3/RConn1 -- Voltage Sensor1/RConn2
  Conn2/RConn1 -- Voltage Sensor1/LConn1
  Conn1/RConn1 -- Voltage Sensor1/RConn1

== system HEV_Battery_Lib/Cells/Subsystem1 ==
  Current Sensor : fl_lib/Electrical/Electrical Sensors/Current Sensor
  Conn1 : PMIOPort  Side=Left
  Conn3 : PMIOPort  Port=2  Side=Right
  Conn2 : PMIOPort  Port=3  Side=Right
  connections:
  Conn3/RConn1 -- Current Sensor/RConn2
  Conn2/RConn1 -- Current Sensor/RConn1
  Conn1/RConn1 -- Current Sensor/LConn1

== system HEV_Battery_Lib/Generic/Measurements ==
  Bus Creator : BusCreator  Inputs=4
  Calc Pct : Gain  Gain=1/HEV_Param.Battery_Sys.Maximum_Capacity*100
  Calculate battery power & charge : Subsystem
  PS-Simulink Converter1 : nesl_utility/PS-Simulink Converter  PhysicalDomain=network_engine_domain  SubClassName=ps_output  LeftPortType=input  RightPortType=output  PseudoPeriodic=off  Frequencies=[]  VectorFormat=1-D array  Unit=V  AffineConversion=off
  PS-Simulink Converter2 : nesl_utility/PS-Simulink Converter  PhysicalDomain=network_engine_domain  SubClassName=ps_output  LeftPortType=input  RightPortType=output  PseudoPeriodic=off  Frequencies=[]  VectorFormat=1-D array  Unit=A  AffineConversion=off
  VBatt : PMIOPort  Side=Left
  IBatt : PMIOPort  Port=2  Side=Left
  Batt_Ah : Outport  VectorParamsAs1DForOutWhenUnconnected=off
  Batt_Meas : Outport  Port=2  VectorParamsAs1DForOutWhenUnconnected=off
  tag scope: Batt_Measures=global
  wires:
  Calculate battery power & charge/1(Ah) -> Bus Creator/1, Calc Pct/1, Batt_Ah/1  "Batt_Ah"
  Calc Pct/1 -> Bus Creator/2  "SOC (%)"
  PS-Simulink Converter1/1 -> Bus Creator/3  "Voltage (V)"
  PS-Simulink Converter2/1 -> Bus Creator/4  "Current (A)"
  Bus Creator/1 -> [Batt_Measures], Batt_Meas/1
  connections:
  Calculate battery power & charge/LConn1 -- VBatt/RConn1 -- PS-Simulink Converter1/LConn1
  Calculate battery power & charge/LConn2 -- IBatt/RConn1 -- PS-Simulink Converter2/LConn1

== system HEV_Battery_Lib/Generic1/Measurements ==
  Bus Creator : BusCreator  Inputs=4
  Calc Pct : Gain  Gain=1/HEV_Param.Battery_Sys.Maximum_Capacity*100
  Calculate battery power & charge : Subsystem
  PS-Simulink Converter1 : nesl_utility/PS-Simulink Converter  PhysicalDomain=network_engine_domain  SubClassName=ps_output  LeftPortType=input  RightPortType=output  PseudoPeriodic=off  Frequencies=[]  VectorFormat=1-D array  Unit=V  AffineConversion=off
  PS-Simulink Converter2 : nesl_utility/PS-Simulink Converter  PhysicalDomain=network_engine_domain  SubClassName=ps_output  LeftPortType=input  RightPortType=output  PseudoPeriodic=off  Frequencies=[]  VectorFormat=1-D array  Unit=A  AffineConversion=off
  VBatt : PMIOPort  Side=Left
  IBatt : PMIOPort  Port=2  Side=Left
  Batt_Ah : Outport  VectorParamsAs1DForOutWhenUnconnected=off
  Batt_Meas : Outport  Port=2  VectorParamsAs1DForOutWhenUnconnected=off
  tag scope: Batt_Measures=global
  wires:
  Calculate battery power & charge/1(Ah) -> Bus Creator/1, Calc Pct/1, Batt_Ah/1  "Batt_Ah"
  Calc Pct/1 -> Bus Creator/2  "SOC (%)"
  PS-Simulink Converter1/1 -> Bus Creator/3  "Voltage (V)"
  PS-Simulink Converter2/1 -> Bus Creator/4  "Current (A)"
  Bus Creator/1 -> [Batt_Measures], Batt_Meas/1
  connections:
  Calculate battery power & charge/LConn1 -- VBatt/RConn1 -- PS-Simulink Converter1/LConn1
  Calculate battery power & charge/LConn2 -- IBatt/RConn1 -- PS-Simulink Converter2/LConn1

== system HEV_Battery_Lib/Predefined/GF1 ==
  In1 : Inport
  SOC Offset : Subsystem
      mask Display: disp('A')
  Out1 : Outport  VectorParamsAs1DForOutWhenUnconnected=off
  tag scope: Batt_Measures=global
  wires:
  SOC Offset/1(Out1) -> Out1/1, [Batt_Measures]
  In1/1 -> SOC Offset/1(In1)

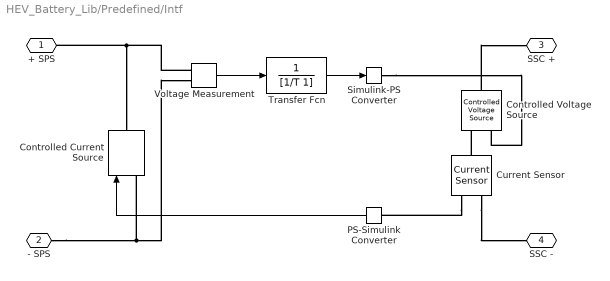
== system HEV_Battery_Lib/Predefined/Intf ==
  Controlled Voltage Source : fl_lib/Electrical/Electrical Sources/Controlled Voltage Source
  Controlled Current Source : spsControlledCurrentSourceLib/Controlled Current Source  Initialize=on  Source_Type=AC  Amplitude=0  Phase=0  Frequency=0  Measurements=None
  Current Sensor : fl_lib/Electrical/Electrical Sensors/Current Sensor
  PS-Simulink Converter : nesl_utility/PS-Simulink Converter  PhysicalDomain=network_engine_domain  SubClassName=ps_output  LeftPortType=input  RightPortType=output  PseudoPeriodic=off  Frequencies=[]  VectorFormat=1-D array  Unit=A  AffineConversion=off
  Simulink-PS Converter : nesl_utility/Simulink-PS Converter  PhysicalDomain=network_engine_domain  SubClassName=ps_input  LeftPortType=input  RightPortType=output  PseudoPeriodic=off  Frequencies=[]  NoiseDistribution=none  NoiseParameters=[]  Unit=V  AffineConversion=off  FilteringAndDerivatives=zero  SimscapeFilterOrder=1  InputFilterTimeConstant=0.005  UdotUserProvided=0
  Transfer Fcn : TransferFcn  Denominator=[1/T 1]
  Voltage Measurement : spsVoltageMeasurementLib/Voltage Measurement  PhasorSimulation=off  OutputType=Complex  PSBequivalent=0
  + SPS : PMIOPort  Side=Left
  - SPS : PMIOPort  Port=2  Side=Left
  SSC + : PMIOPort  Port=3  Side=Right
  SSC - : PMIOPort  Port=4  Side=Right
  wires:
  Transfer Fcn/1 -> Simulink-PS Converter/1
  Voltage Measurement/1 -> Transfer Fcn/1
  PS-Simulink Converter/1 -> Controlled Current Source/1
  connections:
  Voltage Measurement/LConn1 -- + SPS/RConn1 -- Controlled Current Source/RConn1
  Current Sensor/RConn2 -- SSC -/RConn1
  - SPS/RConn1 -- Voltage Measurement/LConn2 -- Controlled Current Source/LConn1
  Current Sensor/RConn1 -- PS-Simulink Converter/LConn1
  Simulink-PS Converter/RConn1 -- Controlled Voltage Source/RConn1
  Current Sensor/LConn1 -- Controlled Voltage Source/RConn2
  Controlled Voltage Source/LConn1 -- SSC +/RConn1

== system HEV_Battery_Lib/RCGeneric/Measurements ==
  Bus Creator : BusCreator  Inputs=4
  Calc Pct : Gain  Gain=1/HEV_Param.Battery_Sys.Maximum_Capacity*100
  Calculate battery power & charge : Subsystem
  PS-Simulink Converter1 : nesl_utility/PS-Simulink Converter  PhysicalDomain=network_engine_domain  SubClassName=ps_output  LeftPortType=input  RightPortType=output  PseudoPeriodic=off  Frequencies=[]  VectorFormat=1-D array  Unit=V  AffineConversion=off
  PS-Simulink Converter2 : nesl_utility/PS-Simulink Converter  PhysicalDomain=network_engine_domain  SubClassName=ps_output  LeftPortType=input  RightPortType=output  PseudoPeriodic=off  Frequencies=[]  VectorFormat=1-D array  Unit=A  AffineConversion=off
  VBatt : PMIOPort  Side=Left
  IBatt : PMIOPort  Port=2  Side=Left
  Batt_Ah : Outport  VectorParamsAs1DForOutWhenUnconnected=off
  Batt_Meas : Outport  Port=2  VectorParamsAs1DForOutWhenUnconnected=off
  tag scope: Batt_Measures=global
  wires:
  Calculate battery power & charge/1(Ah) -> Bus Creator/1, Calc Pct/1, Batt_Ah/1  "Batt_Ah"
  Calc Pct/1 -> Bus Creator/2  "SOC (%)"
  PS-Simulink Converter1/1 -> Bus Creator/3  "Voltage (V)"
  PS-Simulink Converter2/1 -> Bus Creator/4  "Current (A)"
  Bus Creator/1 -> [Batt_Measures], Batt_Meas/1
  connections:
  Calculate battery power & charge/LConn1 -- VBatt/RConn1 -- PS-Simulink Converter1/LConn1
  Calculate battery power & charge/LConn2 -- IBatt/RConn1 -- PS-Simulink Converter2/LConn1

== system HEV_Battery_Lib/Cells/Battery cell1/Thermal Model ==
  Battery thermal mass : fl_lib/Thermal/Thermal Elements/Thermal Mass  mass_type=foundation.enum.constant_variable.constant  mass=1 kg  sp_heat=HEV_Param.Battery_Cell.Ctheta J/kg/K  mass_min=1e-6 kg  num_ports=foundation.enum.numPorts2.one  m_specify=off  m_priority=High  m=1 kg  m_nominal_specify=off  m_nominal_value=1  m_nominal_unit=kg  T_specify=on  T_priority=High  T=HEV_Param.Battery_Cell.theta_init+273 K  T_nominal_specify=off  T_nominal_value=1  T_nominal_unit=K  Q_specify=off  Q_priority=High  Q=0 J/s  Q_nominal_specify=off  Q_nominal_value=1  Q_nominal_unit=J/s
  Ideal Temperature Sensor : fl_lib/Thermal/Thermal Sensors/Temperature Sensor  temperature_measure=foundation.enum.MeasurementReference.difference
  Ideal Heat Flow Source : fl_lib/Thermal/Thermal Sources/Controlled Heat Flow Rate Source
  Kt as a function of temperature : fl_lib/Physical Signals/Lookup Tables/PS Lookup Table (1D)  x=[HEV_Param.Battery_Cell.theta_f,HEV_Param.Battery_Cell. Kt_Temps]+273 K  f=[0 HEV_Param.Battery_Cell.Kt]  interp_method=simscape.enum.interpolation.linear  extrap_method=simscape.enum.extrapolation.linear
  Thermal Reference1 : fl_lib/Thermal/Thermal Elements/Thermal Reference
  Thermal Reference2 : fl_lib/Thermal/Thermal Elements/Thermal Reference
  Ps : PMIOPort  Tag=PMCPort  Side=Left
  H : PMIOPort  Tag=PMCPort  Port=2  Side=Left
  Kt : PMIOPort  Tag=PMCPort  Port=3  Side=Right
  T : PMIOPort  Tag=PMCPort  Port=4  Side=Right
  connections:
  Ideal Temperature Sensor/RConn1 -- Thermal Reference2/LConn1
  Ideal Temperature Sensor/RConn2 -- Kt as a function of temperature/LConn1 -- T/RConn1
  Thermal Reference1/LConn1 -- Ideal Heat Flow Source/RConn2
  H/RConn1 -- Ideal Temperature Sensor/LConn1 -- Ideal Heat Flow Source/LConn1 -- Battery thermal mass/LConn1
  Kt/RConn1 -- Kt as a function of temperature/RConn1
  Ideal Heat Flow Source/RConn1 -- Ps/RConn1

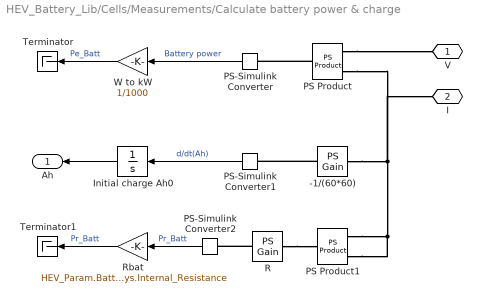
== system HEV_Battery_Lib/Cells/Measurements/Calculate battery power & charge ==
  -1/(60*60) : fl_lib/Physical Signals/Functions/PS Gain  gain=-1/(60*60)
  Initial charge Ah0 : Integrator  InitialCondition=HEV_Param.Battery_Sys.Maximum_Capacity
  PS Product : fl_lib/Physical Signals/Functions/PS Product
  PS Product1 : fl_lib/Physical Signals/Functions/PS Product
  PS-Simulink Converter : nesl_utility/PS-Simulink Converter  PhysicalDomain=network_engine_domain  SubClassName=ps_output  LeftPortType=input  RightPortType=output  PseudoPeriodic=off  Frequencies=[]  VectorFormat=1-D array  Unit=W  AffineConversion=off
  PS-Simulink Converter1 : nesl_utility/PS-Simulink Converter  PhysicalDomain=network_engine_domain  SubClassName=ps_output  LeftPortType=input  RightPortType=output  PseudoPeriodic=off  Frequencies=[]  VectorFormat=1-D array  Unit=A  AffineConversion=off
  PS-Simulink Converter2 : nesl_utility/PS-Simulink Converter  PhysicalDomain=network_engine_domain  SubClassName=ps_output  LeftPortType=input  RightPortType=output  PseudoPeriodic=off  Frequencies=[]  VectorFormat=1-D array  Unit=W  AffineConversion=off
  R : fl_lib/Physical Signals/Functions/PS Gain  gain=HEV_Param.Battery_Sys.Internal_Resistance Ohm
  Rbat : Gain  Gain=HEV_Param.Battery_Sys.Internal_Resistance
  Terminator : Terminator
  Terminator1 : Terminator
  W to kW : Gain  Gain=1/1000
  V : PMIOPort  Side=Left
  I : PMIOPort  Port=2  Side=Left
  Ah : Outport  VectorParamsAs1DForOutWhenUnconnected=off
  wires:
  Rbat/1 -> Terminator1/1  "Pr_Batt"
  Initial charge Ah0/1 -> Ah/1
  W to kW/1 -> Terminator/1  "Pe_Batt"
  PS-Simulink Converter1/1 -> Initial charge Ah0/1  "d/dt(Ah)"
  PS-Simulink Converter2/1 -> Rbat/1  "Pr_Batt"
  PS-Simulink Converter/1 -> W to kW/1  "Battery power"
  connections:
  -1/(60*60)/LConn1 -- PS Product/LConn2 -- I/RConn1 -- PS Product1/LConn2 -- PS Product1/LConn1
  PS Product/LConn1 -- V/RConn1
  R/LConn1 -- PS Product1/RConn1
  -1/(60*60)/RConn1 -- PS-Simulink Converter1/LConn1
  R/RConn1 -- PS-Simulink Converter2/LConn1
  PS Product/RConn1 -- PS-Simulink Converter/LConn1

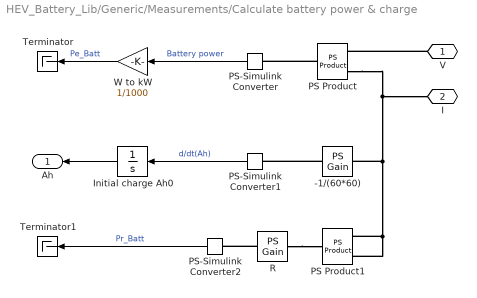
== system HEV_Battery_Lib/Generic/Measurements/Calculate battery power & charge ==
  -1/(60*60) : fl_lib/Physical Signals/Functions/PS Gain  gain=-1/(60*60)
  Initial charge Ah0 : Integrator  InitialCondition=HEV_Param.Battery_Sys.Maximum_Capacity
  PS Product : fl_lib/Physical Signals/Functions/PS Product
  PS Product1 : fl_lib/Physical Signals/Functions/PS Product
  PS-Simulink Converter : nesl_utility/PS-Simulink Converter  PhysicalDomain=network_engine_domain  SubClassName=ps_output  LeftPortType=input  RightPortType=output  PseudoPeriodic=off  Frequencies=[]  VectorFormat=1-D array  Unit=W  AffineConversion=off
  PS-Simulink Converter1 : nesl_utility/PS-Simulink Converter  PhysicalDomain=network_engine_domain  SubClassName=ps_output  LeftPortType=input  RightPortType=output  PseudoPeriodic=off  Frequencies=[]  VectorFormat=1-D array  Unit=A  AffineConversion=off
  PS-Simulink Converter2 : nesl_utility/PS-Simulink Converter  PhysicalDomain=network_engine_domain  SubClassName=ps_output  LeftPortType=input  RightPortType=output  PseudoPeriodic=off  Frequencies=[]  VectorFormat=1-D array  Unit=W  AffineConversion=off
  R : fl_lib/Physical Signals/Functions/PS Gain  gain=HEV_Param.Battery_Sys.Internal_Resistance Ohm
  Terminator : Terminator
  Terminator1 : Terminator
  W to kW : Gain  Gain=1/1000
  V : PMIOPort  Side=Left
  I : PMIOPort  Port=2  Side=Left
  Ah : Outport  VectorParamsAs1DForOutWhenUnconnected=off
  wires:
  PS-Simulink Converter/1 -> W to kW/1  "Battery power"
  W to kW/1 -> Terminator/1  "Pe_Batt"
  PS-Simulink Converter1/1 -> Initial charge Ah0/1  "d/dt(Ah)"
  Initial charge Ah0/1 -> Ah/1
  PS-Simulink Converter2/1 -> Terminator1/1  "Pr_Batt"
  connections:
  R/RConn1 -- PS-Simulink Converter2/LConn1
  PS Product/RConn1 -- PS-Simulink Converter/LConn1
  V/RConn1 -- PS Product/LConn1
  PS Product/LConn2 -- I/RConn1 -- -1/(60*60)/LConn1 -- PS Product1/LConn1 -- PS Product1/LConn2
  -1/(60*60)/RConn1 -- PS-Simulink Converter1/LConn1
  R/LConn1 -- PS Product1/RConn1

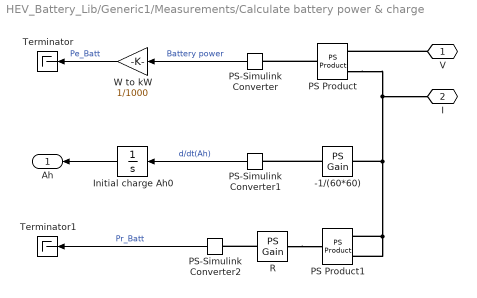
== system HEV_Battery_Lib/Generic1/Measurements/Calculate battery power & charge ==
  -1/(60*60) : fl_lib/Physical Signals/Functions/PS Gain  gain=-1/(60*60)
  Initial charge Ah0 : Integrator  InitialCondition=HEV_Param.Battery_Sys.Maximum_Capacity
  PS Product : fl_lib/Physical Signals/Functions/PS Product
  PS Product1 : fl_lib/Physical Signals/Functions/PS Product
  PS-Simulink Converter : nesl_utility/PS-Simulink Converter  PhysicalDomain=network_engine_domain  SubClassName=ps_output  LeftPortType=input  RightPortType=output  PseudoPeriodic=off  Frequencies=[]  VectorFormat=1-D array  Unit=W  AffineConversion=off
  PS-Simulink Converter1 : nesl_utility/PS-Simulink Converter  PhysicalDomain=network_engine_domain  SubClassName=ps_output  LeftPortType=input  RightPortType=output  PseudoPeriodic=off  Frequencies=[]  VectorFormat=1-D array  Unit=A  AffineConversion=off
  PS-Simulink Converter2 : nesl_utility/PS-Simulink Converter  PhysicalDomain=network_engine_domain  SubClassName=ps_output  LeftPortType=input  RightPortType=output  PseudoPeriodic=off  Frequencies=[]  VectorFormat=1-D array  Unit=W  AffineConversion=off
  R : fl_lib/Physical Signals/Functions/PS Gain  gain=HEV_Param.Battery_Sys.Internal_Resistance Ohm
  Terminator : Terminator
  Terminator1 : Terminator
  W to kW : Gain  Gain=1/1000
  V : PMIOPort  Side=Left
  I : PMIOPort  Port=2  Side=Left
  Ah : Outport  VectorParamsAs1DForOutWhenUnconnected=off
  wires:
  PS-Simulink Converter/1 -> W to kW/1  "Battery power"
  W to kW/1 -> Terminator/1  "Pe_Batt"
  PS-Simulink Converter1/1 -> Initial charge Ah0/1  "d/dt(Ah)"
  Initial charge Ah0/1 -> Ah/1
  PS-Simulink Converter2/1 -> Terminator1/1  "Pr_Batt"
  connections:
  R/RConn1 -- PS-Simulink Converter2/LConn1
  PS Product/RConn1 -- PS-Simulink Converter/LConn1
  V/RConn1 -- PS Product/LConn1
  PS Product/LConn2 -- I/RConn1 -- -1/(60*60)/LConn1 -- PS Product1/LConn1 -- PS Product1/LConn2
  -1/(60*60)/RConn1 -- PS-Simulink Converter1/LConn1
  R/LConn1 -- PS Product1/RConn1
